simulink model "sim_observer"  (R2017a)
settings: Solver=VariableStepAuto  StartTime=0.0  StopTime=10.0  RelTol=1e-3
values from neighbouring files (symbols this model uses):
  a_k = 1/(size(A,1)+1)    [Init.m]
  x0 = reshape(x0_d,[],1)    [Init.m]
settings Model: Creator=Piotr Chudalewski  LastModifiedBy=Piotr Chudalewski

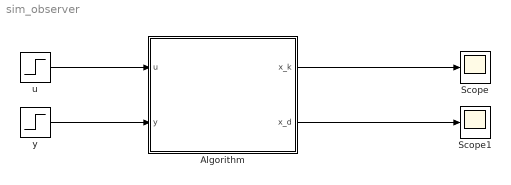
== system sim_observer ==
  Algorithm : Subsystem  mask{A=[ 1 1; 0 1], B=[2;3], C=[1 3], L=[-13;6]}
      mask prompts: A "Matrix A"; B "Matrix B"; C "Matrix C"; L "Matrix L"
      mask init:
      | Init
  Scope : Scope
  Scope1 : Scope
  u : Step  Before=[0 ;0; 0]  SampleTime=0
  y : Step  Before=[0;0;0]  SampleTime=0
  wires:
  u/1 -> Algorithm/1(u)
  Algorithm/1(x_k) -> Scope/1
  y/1 -> Algorithm/2(y)
  Algorithm/2(x_d) -> Scope1/1

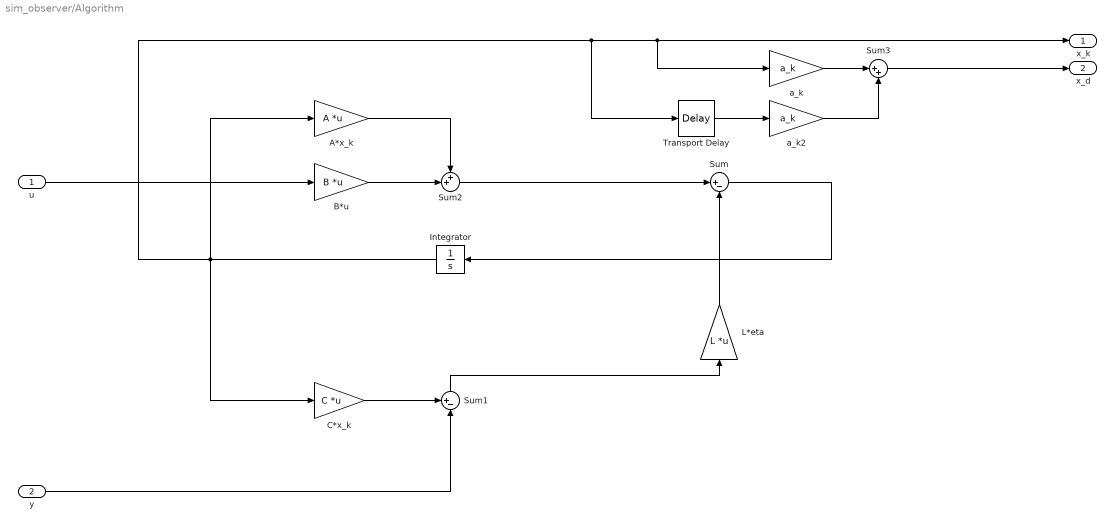
== system sim_observer/Algorithm ==
  u : Inport
  y : Inport  Port=2
  A*x_k : Gain  Gain=A  Multiplication=Matrix(K*u)
  B*u : Gain  Gain=B  Multiplication=Matrix(K*u)
  C*x_k : Gain  Gain=C  Multiplication=Matrix(K*u)
  Integrator : Integrator  InitialCondition=x0
  "L*eta " : Gain  Gain=L  Multiplication=Matrix(K*u)
  Sum : Sum  Inputs=|+-
  Sum1 : Sum  Inputs=+-|
  Sum2 : Sum  Inputs=++|
  Sum3 : Sum  Inputs=|++
  Transport Delay : TransportDelay  DelayTime=0.5
  a_k : Gain  Gain=a_k
  a_k2 : Gain  Gain=a_k
  x_k : Outport
  x_d : Outport  Port=2
  wires:
  Sum/1 -> Integrator/1
  Sum1/1 -> "L*eta "/1
  Sum2/1 -> Sum/1
  u/1 -> B*u/1
  y/1 -> Sum1/2
  C*x_k/1 -> Sum1/1
  "L*eta "/1 -> Sum/2
  A*x_k/1 -> Sum2/1
  B*u/1 -> Sum2/2
  Integrator/1 -> C*x_k/1, a_k/1, x_k/1, Transport Delay/1, A*x_k/1
  Sum3/1 -> x_d/1
  a_k/1 -> Sum3/1
  a_k2/1 -> Sum3/2
  Transport Delay/1 -> a_k2/1
